simulink model "Untitled1"  (R2014a)
settings: Solver=ode45  StartTime=0.0  StopTime=10.0  RelTol=1e-3
values from neighbouring files (symbols this model uses):
  Ad = [ -0.6 0 0; 0.02 -0.8 0;0  0 0.3 ;]    [Lab4.m]    (also in online_1.m = Omegam(1:3,1:3))
  Bd = [ -2; 1; 2 ]    [Lab4.m]    (also in online_1.m = Omegam(4,:))
  Dd = 0    [Lab4.m]
undefined symbols (not defined in the file or in its folder): C
settings Model: Creator=pal.janos-attila  LastModifiedBy=pal.janos-attila

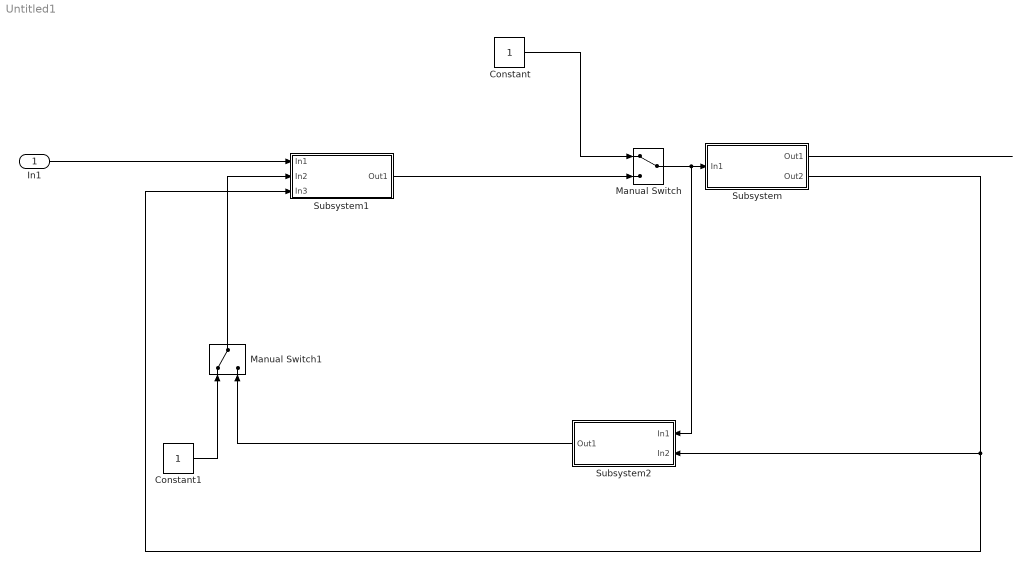
== system Untitled1 ==
  In1 : Inport
  Constant : Constant
  Constant1 : Constant
  Manual Switch : ManualSwitch
  Manual Switch1 : ManualSwitch
  Subsystem : Subsystem
  Subsystem1 : Subsystem
  Subsystem2 : Subsystem
  wires:
  Constant/1 -> Manual Switch/1
  Constant1/1 -> Manual Switch1/1
  Subsystem1/1(Out1) -> Manual Switch/2
  Manual Switch1/1 -> Subsystem1/2(In2)
  In1/1 -> Subsystem1/1(In1)
  Subsystem/1(Out1) -> ?
  Subsystem2/1(Out1) -> Manual Switch1/2
  Subsystem/2(Out2) -> Subsystem2/2(In2), Subsystem1/3(In3)
  Manual Switch/1 -> Subsystem2/1(In1), Subsystem/1(In1)

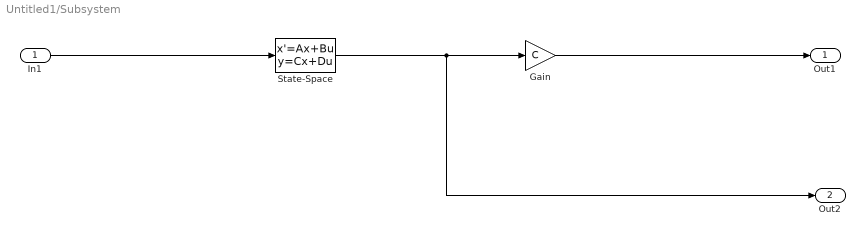
== system Untitled1/Subsystem ==
  In1 : Inport
  Gain : Gain  Gain=C
  State-Space : StateSpace  A=Ad  B=Bd  C=eye(3)  D=Dd  X0=0
  Out1 : Outport
  Out2 : Outport  Port=2
  wires:
  In1/1 -> State-Space/1
  State-Space/1 -> Out2/1, Gain/1
  Gain/1 -> Out1/1

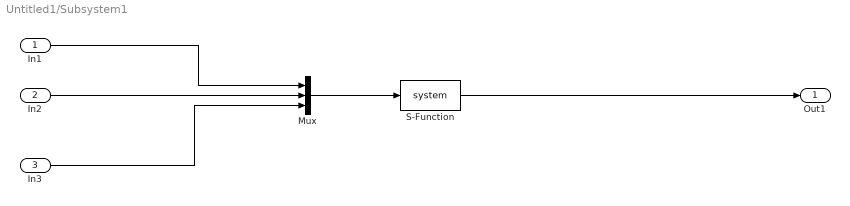
== system Untitled1/Subsystem1 ==
  In1 : Inport
  In2 : Inport  Port=2
  In3 : Inport  Port=3
  Mux : Mux  Inputs=3
  S-Function : S-Function  EnableBusSupport=off
  Out1 : Outport
  wires:
  S-Function/1 -> Out1/1
  Mux/1 -> S-Function/1
  In1/1 -> Mux/1
  In2/1 -> Mux/2
  In3/1 -> Mux/3

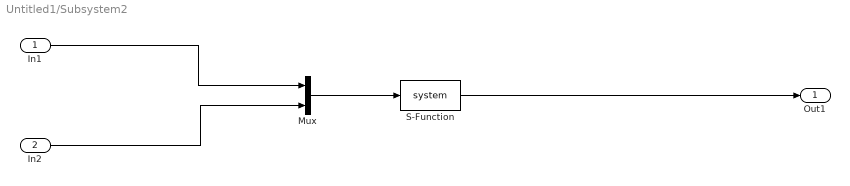
== system Untitled1/Subsystem2 ==
  In1 : Inport
  In2 : Inport  Port=2
  Mux : Mux  Inputs=2
  S-Function : S-Function  EnableBusSupport=off
  Out1 : Outport
  wires:
  S-Function/1 -> Out1/1
  Mux/1 -> S-Function/1
  In1/1 -> Mux/1
  In2/1 -> Mux/2
